simulink library "INP_IMU_EB"  (R2023b)
settings: Solver=VariableStepAuto  StartTime=0.0  StopTime=10.0  RelTol=1e-3
libraries: INP_IMU_Prep_EB x1, INP_IMU_ManOver_EB x1, INP_IMU_Comp_EB x1
settings Model: Creator=blatak  LastModifiedBy=blatak

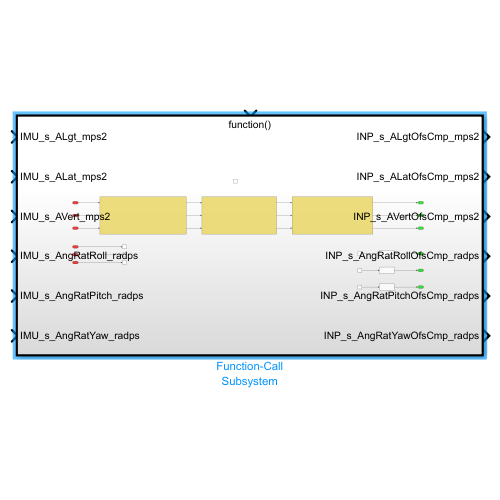
[thumbnail: Simulink's stored preview of the top-level diagram]
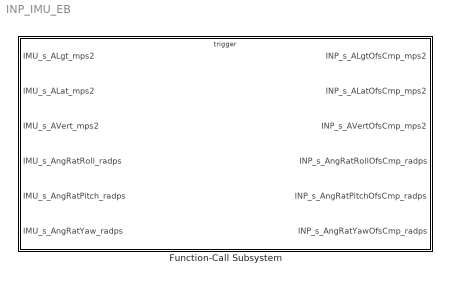
== system INP_IMU_EB ==
  Function-Call Subsystem : Subsystem  TreatAsAtomicUnit=on

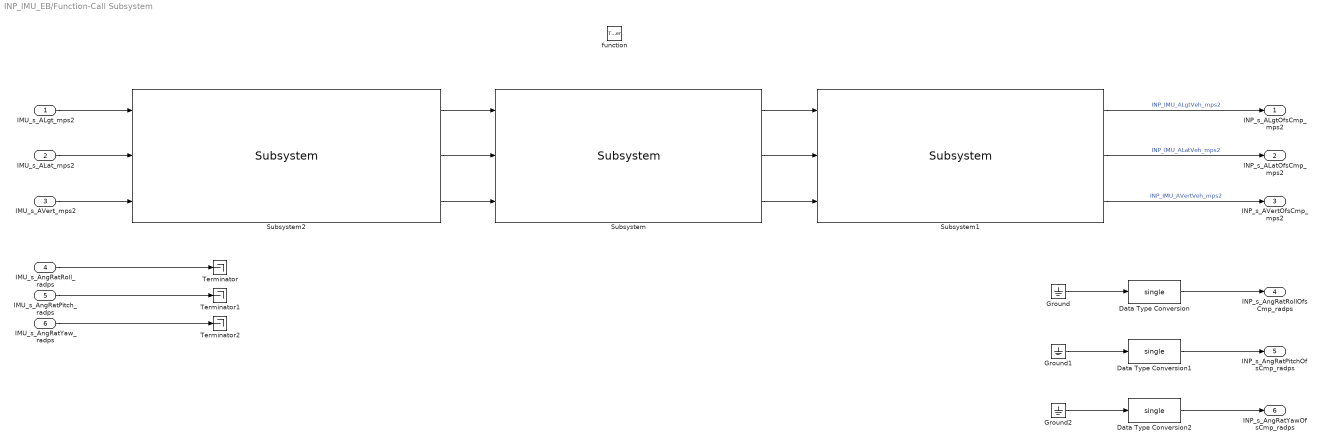
== system INP_IMU_EB/Function-Call Subsystem ==
  IMU_s_ALgt_mps2 : Inport
  IMU_s_ALat_mps2 : Inport  Port=2
  IMU_s_AVert_mps2 : Inport  Port=3
  IMU_s_AngRatRoll_radps : Inport  Port=4
  IMU_s_AngRatPitch_radps : Inport  Port=5
  IMU_s_AngRatYaw_radps : Inport  Port=6
  function : TriggerPort  TriggerType=function-call  VariantControl=(inherit)
  Data Type Conversion : DataTypeConversion  OutDataTypeStr=single  SaturateOnIntegerOverflow=off  RndMeth=Floor
  Data Type Conversion1 : DataTypeConversion  OutDataTypeStr=single  SaturateOnIntegerOverflow=off  RndMeth=Floor
  Data Type Conversion2 : DataTypeConversion  OutDataTypeStr=single  SaturateOnIntegerOverflow=off  RndMeth=Floor
  Ground : Ground
  Ground1 : Ground
  Ground2 : Ground
  Subsystem : INP_IMU_Prep_EB/Subsystem  SystemSampleTime=-1  VariantActivationTime=update diagram  AllowFlexibleInterface=on  Latency=0  AutoFrameSizeCalculation=off
  Subsystem1 : INP_IMU_ManOver_EB/Subsystem  SystemSampleTime=-1  VariantActivationTime=update diagram  AllowFlexibleInterface=on  Latency=0  AutoFrameSizeCalculation=off
  Subsystem2 : INP_IMU_Comp_EB/Subsystem  SystemSampleTime=-1  VariantActivationTime=update diagram  AllowFlexibleInterface=on  Latency=0  AutoFrameSizeCalculation=off
  Terminator : Terminator
  Terminator1 : Terminator
  Terminator2 : Terminator
  INP_s_ALgtOfsCmp_mps2 : Outport
  INP_s_ALatOfsCmp_mps2 : Outport  Port=2
  INP_s_AVertOfsCmp_mps2 : Outport  Port=3
  INP_s_AngRatRollOfsCmp_radps : Outport  Port=4
  INP_s_AngRatPitchOfsCmp_radps : Outport  Port=5
  INP_s_AngRatYawOfsCmp_radps : Outport  Port=6
  wires:
  Data Type Conversion2/1 -> INP_s_AngRatYawOfsCmp_radps/1
  Data Type Conversion1/1 -> INP_s_AngRatPitchOfsCmp_radps/1
  Subsystem1/1 -> INP_s_ALgtOfsCmp_mps2/1  "INP_IMU_ALgtVeh_mps2"
  Data Type Conversion/1 -> INP_s_AngRatRollOfsCmp_radps/1
  Subsystem1/3 -> INP_s_AVertOfsCmp_mps2/1  "INP_IMU_AVertVeh_mps2"
  Subsystem1/2 -> INP_s_ALatOfsCmp_mps2/1  "INP_IMU_ALatVeh_mps2"
  IMU_s_AngRatRoll_radps/1 -> Terminator/1
  IMU_s_ALgt_mps2/1 -> Subsystem2/1
  IMU_s_ALat_mps2/1 -> Subsystem2/2
  IMU_s_AngRatPitch_radps/1 -> Terminator1/1
  IMU_s_AngRatYaw_radps/1 -> Terminator2/1
  IMU_s_AVert_mps2/1 -> Subsystem2/3
  Subsystem2/1 -> Subsystem/1
  Subsystem2/2 -> Subsystem/2
  Subsystem2/3 -> Subsystem/3
  Subsystem/1 -> Subsystem1/1
  Subsystem/2 -> Subsystem1/2
  Subsystem/3 -> Subsystem1/3
  Ground/1 -> Data Type Conversion/1
  Ground2/1 -> Data Type Conversion2/1
  Ground1/1 -> Data Type Conversion1/1
